simulink model "data_visualization"  (R2023b)
settings: Solver=ode3  StartTime=0.0  StopTime=100  RelTol=1e-3  EnableMultiTasking=on
undefined symbols (not defined in the file): LF
libraries: simulink_extras x3, instrumentseriallib x2, sim3dlib x1, uavsim3dlib x1
settings Model: FPTRunName=Active  ExtModeTrigDuration=2  Creator=kikip  LastModifiedBy=kikip
settings SolverCC: AlgebraicLoopSolver=TrustRegion  AutoInsertRateTranBlk=on
settings DataIOCC: LimitDataPoints=on  SaveFormat=Array
settings OptimizationCC: ReuseModelBlockBuffer=off  ExpressionDepthLimit=2147483647  LifeSpan=Inf  MaxStackSize=64
settings DebuggingCC: UnderspecifiedInitializationDetection=Classic  MergeDetectMultiDrivingBlocksExec=none  FcnCallInpInsideContextMsg=warning  UnconnectedInputMsg=warning  UnconnectedOutputMsg=warning  UnconnectedLineMsg=warning  AllowSymbolicDim=off  StateNameClashWarn=warning  SFUnexpectedBacktrackingDiag=warning  SFNoUnconditionalDefaultTransitionDiag=warning  SFExecutionAtInitializationDiag=none  ArithmeticOperatorsInVariantConditions=warning
settings HardwareCC: ProdBitPerPointer=32  ProdBitPerSizeT=32  ProdBitPerPtrDiffT=32  ProdLargestAtomicInteger=Long  ProdLargestAtomicFloat=Double  ProdWordSize=32  ProdHWDeviceType=ARM Compatible->ARM Cortex  UseEmbeddedCoderFeatures=off  UseSimulinkCoderFeatures=off
settings ModelReferenceCC: EnableRefExpFcnMdlSchedulingChecks=on  PropagateSignalLabelsOutOfModel=off
settings SFSimCC: SimUseLocalCustomCode=off  CustomCodeUndefinedFunction=UseInterfaceOnly
settings RTWCC: Description=Embedded Coder  SystemTargetFile=ert.tlc  HardwareBoard=ESP32-WROOM(Arduino Compatible)  TemplateMakefile=ert_default_tmf  GenerateReport=on  RTWVerbose=off  RTWUseLocalCustomCode=off  Toolchain=ESP32  BuildConfiguration=Faster Runs  LaunchReport=on
settings CodeAppCC: ForceParamTrailComments=on  OperatorAnnotations=on  StateflowObjectComments=on  MATLABSourceComments=on
settings ERTTargetCC: MultiwordLength=2048  ERTCustomFileBanners=off  SupportContinuousTime=on  SupportNonInlinedSFcns=on  RemoveResetFunc=off  SupportVariableSizeSignals=on  ModelStepFunctionPrototypeControlCompliant=off  ExtModeTransport=3  ExtModeStaticAlloc=on  ExtModeAutomaticAllocSize=off  ExtModeStaticAllocSize=65536  ExtModeMexFile=ext_xcp  ExtModeIntrfLevel=Level2 - Open
settings ConfigComp: CovMetricSettings=dw  CovSaveCumulativeToWorkspaceVar=on  CovSaveSingleToWorkspaceVar=on  CovExternalEMLEnable=off  CovSFcnEnable=off

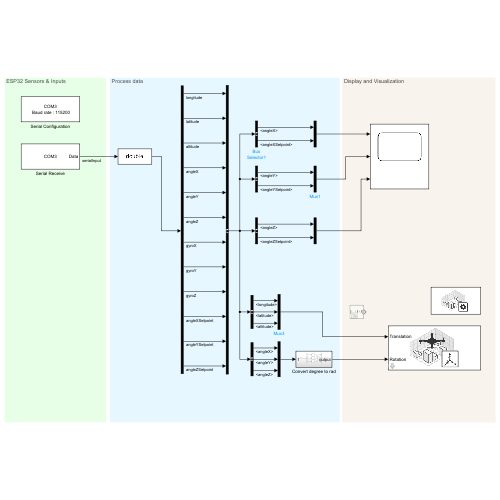
[thumbnail: Simulink's stored preview of the top-level diagram]
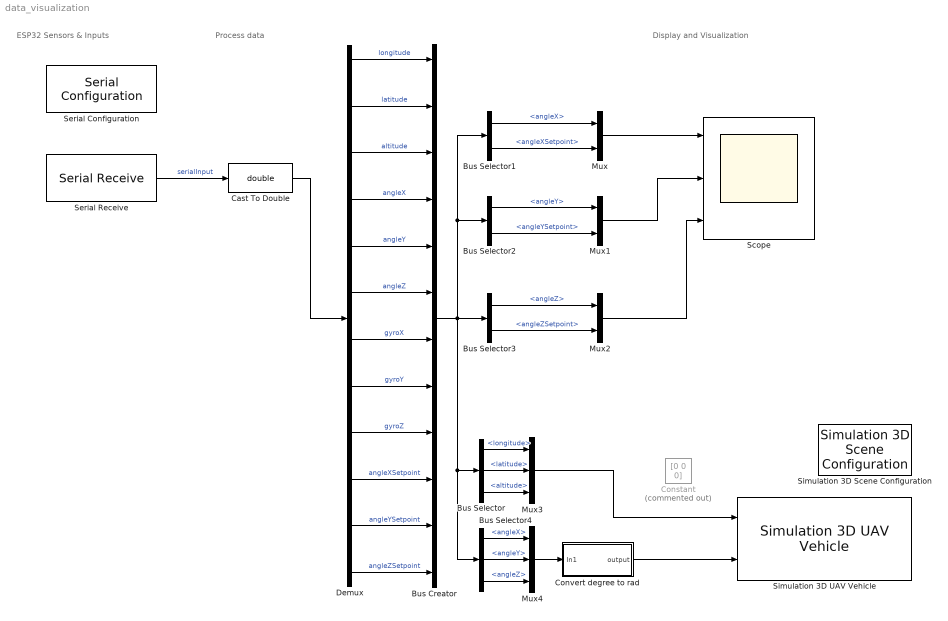
== system data_visualization ==
  note: Display and Visualization
  note: ESP32 Sensors & Inputs
  note: Process data
  Bus Creator : BusCreator  Inputs=12
  Bus Selector : BusSelector  OutputSignals=longitude,latitude,altitude
  Bus Selector1 : BusSelector  OutputSignals=angleX,angleXSetpoint
  Bus Selector2 : BusSelector  OutputSignals=angleY,angleYSetpoint
  Bus Selector3 : BusSelector  OutputSignals=angleZ,angleZSetpoint
  Bus Selector4 : BusSelector  OutputSignals=angleX,angleY,angleZ
  Cast To Double : DataTypeConversion  OutDataTypeStr=double  SaturateOnIntegerOverflow=off  RndMeth=Floor
  Constant : Constant  Commented=on  Value=[0 0 0]
  Convert degree to rad : Subsystem
  Demux : Demux  Outputs=12
  Mux : Mux  Inputs=2
  Mux1 : Mux  Inputs=2
  Mux2 : Mux  Inputs=2
  Mux3 : Mux  Inputs=3
  Mux4 : Mux  Inputs=3
  Scope : Scope  NumInputPorts=3
  Serial Configuration : instrumentseriallib/Serial Configuration  Priority=-200000  PortSel=COM3  Port=COM3  ComPort=COM3  BaudRate=115200  DataBits=8  Parity=none  StopBits=1  ByteOrder=little-endian  FlowControl=none  Timeout=10  SimulateUsing=Interpreted execution  BlockInModel=on  aMode=1
  Serial Receive : instrumentseriallib/Serial Receive  Priority=1  PortSel=COM3  Port=COM3  ComPort=COM3  DataType=single  SaveDataType=uint8  ToggleHeader=on  Header='A'  ToggleTerminator=on  Terminator=LF ('\n')  CustomTerminator=[]  InputFormat=Column major  ToggleDataSize=on  DataSize=[1 12]  EnableBlockingMode=on  ActionDataUnavailable=Output last received value  ActionWhenDataUnavailable=Output last received value  CustomValue=0  SampleTime=0.01  SimulateUsing=Interpreted execution  BlockInModel=on  aMode=1
  Simulation 3D Scene Configuration : sim3dlib/Simulation 3D Scene Configuration  Priority=0  ProjectFormat=Default Scenes  SceneDesc=US city block  ProjectName=E:\MATLAB\R2023b\toolbox\shared\sim3d_projects\automotive_project_windows\UE\WindowsNoEditor\VehicleSimulation.exe  ScenePath=/Game/Maps/USCityBlock  EnableOpenDRIVE=off  vehTagList={'Custom';'Scene Origin';'TeamDragon'}  vehTag=TeamDragon  FreeCameraInitialTranslation=[0, 0, 0]  FreeCameraDefaultInitialTranslation=[-6, 0, 2]  FreeCameraInitialRotation=[0, 0, 0]  FreeCameraDefaultInitialRotation=[0, -15, 0]  OpVisEn=off  Ts=0.05  EnableWindow=on  EnableRemoteAccess=off  EnableWeather=off  SunAltitude=40.0  SunAzimuth=90  clouds=10  wind=1  fog=0  rain=0  EnableGeospatial=off  OriginHeight=200  OriginLatitude=40.744652  OriginLongitude=-73.988864  MapStyle=Aerial  AdditionalAssetIDs=[]  UseAdvancedSunSky=off  SolarTime=11  TimeZone=-5  Day=21  Month=9  Year=2022  UseDaylightSavingTime=on  DSTStartDay=10  DSTStartMonth=3  DSTEndDay=3  DSTEndMonth=11  DSTSwitchHour=2  sensorTag=MainCamera1  sensorId=1  sensorName=MainCamera1  mountLoc=Origin  offsetFlag=off  tmountOffset=[0, 0, 0]  rmountOffset=[0, 0, 0]  HorizontalResolution=1280  VerticalResolution=720  HorizontalFOV=60  mountPoint=[0 0 0]  mountOrientation=[0 0 0]  aMode=4  ID=1  GeoTrigger=Inactive
      settings: LibrarySourceBlock=uavsim3dlib/Simulation 3D Scene Configuration
  Simulation 3D UAV Vehicle : uavsim3dlib/Simulation 3D UAV Vehicle  Priority=-1  Mesh=Quadrotor  MeshPath=/MathWorksUAVContent/UAVs/HexaRotorUAV/HexaRotor.HexaRotor  Color=Silver  ActorName=TeamDragon  UseGlobalFrame=off  InitialTranslation=[0 0 0]  InitialRotation=[0 0 0]  InitialTranslationGlobal=[0 0 0]  InitialGeoOrigin=[0 0 0]  InitialRotationGlobal=[0 0 0]  SampleTime=-1  ActorType=SimulinkVehicle  ID=C  aMode=4  ActorTag=TeamDragon
  wires:
  Serial Receive/1 -> Cast To Double/1  "serialInput"
  Demux/1 -> Bus Creator/1  "longitude"
  Demux/2 -> Bus Creator/2  "latitude"
  Demux/3 -> Bus Creator/3  "altitude"
  Demux/7 -> Bus Creator/7  "gyroX"
  Demux/8 -> Bus Creator/8  "gyroY"
  Demux/9 -> Bus Creator/9  "gyroZ"
  Demux/10 -> Bus Creator/10  "angleXSetpoint"
  Demux/11 -> Bus Creator/11  "angleYSetpoint"
  Demux/12 -> Bus Creator/12  "angleZSetpoint"
  Cast To Double/1 -> Demux/1
  Convert degree to rad/1(output) -> Simulation 3D UAV Vehicle/2
  Bus Selector1/1 -> Mux/1  "<angleX>"
  Bus Selector1/2 -> Mux/2  "<angleXSetpoint>"
  Mux/1 -> Scope/1
  Bus Selector2/1 -> Mux1/1  "<angleY>"
  Bus Selector2/2 -> Mux1/2  "<angleYSetpoint>"
  Mux1/1 -> Scope/2
  Bus Selector3/1 -> Mux2/1  "<angleZ>"
  Mux2/1 -> Scope/3
  Bus Creator/1 -> Bus Selector2/1, Bus Selector1/1, Bus Selector3/1, Bus Selector4/1, Bus Selector/1
  Bus Selector/1 -> Mux3/1  "<longitude>"
  Bus Selector/2 -> Mux3/2  "<latitude>"
  Bus Selector/3 -> Mux3/3  "<altitude>"
  Demux/4 -> Bus Creator/4  "angleX"
  Demux/5 -> Bus Creator/5  "angleY"
  Demux/6 -> Bus Creator/6  "angleZ"
  Bus Selector3/2 -> Mux2/2  "<angleZSetpoint>"
  Mux3/1 -> Simulation 3D UAV Vehicle/1
  Bus Selector4/1 -> Mux4/1  "<angleX>"
  Bus Selector4/3 -> Mux4/3  "<angleZ>"
  Bus Selector4/2 -> Mux4/2  "<angleY>"
  Mux4/1 -> Convert degree to rad/1(In1)

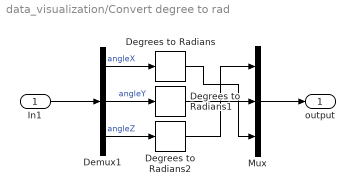
== system data_visualization/Convert degree to rad ==
  In1 : Inport
  Degrees to Radians : simulink_extras/Transformations/Degrees to Radians
  Degrees to Radians1 : simulink_extras/Transformations/Degrees to Radians
  Degrees to Radians2 : simulink_extras/Transformations/Degrees to Radians
  Demux1 : Demux  Outputs=3
  Mux : Mux  Inputs=3
  output : Outport
  wires:
  Demux1/3 -> Degrees to Radians2/1  "angleZ"
  Demux1/2 -> Degrees to Radians1/1  "angleY"
  Demux1/1 -> Degrees to Radians/1  "angleX"
  In1/1 -> Demux1/1
  Degrees to Radians/1 -> Mux/3
  Degrees to Radians1/1 -> Mux/2
  Degrees to Radians2/1 -> Mux/1
  Mux/1 -> output/1
